simulink model "pendoloKalman"  (R2021a)
settings: Solver=VariableStepAuto  StartTime=0.0  StopTime=10.0  RelTol=1e-3
settings Model: Creator=adolfocafaro  LastModifiedBy=adolfocafaro

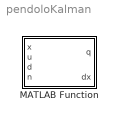
== system pendoloKalman ==
  MATLAB Function : MATLAB Function  TreatAsAtomicUnit=on

== matlab function pendoloKalman/MATLAB Function ==
  data: x input; u input; q output; d input; n input; dx output
function [q,dx] = pendolo(x,u,d,n)
A = [0 1;-g/d 0];
B = [0;1/d^2*m];

Vd=0.1*eye(2); %matrice cov disturbo processo
Vn=1; %matrice cov rumore misurazione

Bd=[B Vd zeros(2,1)];
Dd=[0 0 0 1];

C = [1 0];
U = [u;d;n];

dx = A * x + Bd * U;
q  = C * x + Dd * U;
